simulink model "reaction_pendulum_swingup"  (R2021b)
settings: Solver=FixedStepDiscrete  StartTime=0.0  StopTime=15  FixedStep=h  RelTol=1e-3  EnableMultiTasking=on
PreLoadFcn:
  | warning('off','MATLAB:dispatcher:InexactMatch');
InitFcn:
  | startup_sequence
StartFcn:
  | startup_sequence
model workspace (MAT data in the model file):
  square_freq = 0.5
values from neighbouring files (symbols this model uses):
  F = A22-L*A12    [Reduced_observer.m]
  G = A21-L*A11+F*L    [Reduced_observer.m]
  H = B2-L*B1    [Reduced_observer.m]
  K_LQR = lqr(A,B,Q,R)    [LQR_gain.m]
  L = 10    [LQR_gain.m]    (also in Reduced_observer.m = place(A22',A12',pole)')
  linearization_point = [pi;0;0]    [startup_sequence.m]
  lp_deviation = [deg2rad((rand()-0.5)*50+180);0;0]    [startup_sequence.m]
undefined symbols (not defined in the file or in its folder): DiscIntNeverNeededParam, H_nlobs
settings Model: ExtModeTrigDuration=100000  Creator=user  LastModifiedBy=niels
settings DataIOCC: SaveFormat=Array  SignalLoggingSaveFormat=ModelDataLogs  SaveOutput=off  SignalLogging=off  DSMLogging=off  SaveTime=off  ReturnWorkspaceOutputs=off
settings OptimizationCC: ExpressionDepthLimit=2147483647  LifeSpan=inf
settings DebuggingCC: UnderspecifiedInitializationDetection=Classic  MergeDetectMultiDrivingBlocksExec=none  SolverPrmCheckMsg=warning  FcnCallInpInsideContextMsg=warning  StateNameClashWarn=warning  SFUnexpectedBacktrackingDiag=warning  SFNoUnconditionalDefaultTransitionDiag=warning  SFExecutionAtInitializationDiag=none  ArithmeticOperatorsInVariantConditions=warning
settings HardwareCC: ProdBitPerPointer=32  ProdBitPerSizeT=32  ProdBitPerPtrDiffT=32  ProdLargestAtomicFloat=None  ProdIntDivRoundTo=Undefined  ProdEndianess=Unspecified  ProdWordSize=32  ProdHWDeviceType=32-bit Generic
settings ModelReferenceCC: PropagateSignalLabelsOutOfModel=off
settings SFSimCC: SimUseLocalCustomCode=off  CustomCodeUndefinedFunction=UseInterfaceOnly
settings RTWCC: Description=rpend RTDAC/USB2 (Visual C/C++)  SystemTargetFile=rtcon_rpend_usb2.tlc  TemplateMakefile=rtcon_rpend_vc_usb2_x64.tmf  RTWUseLocalCustomCode=off
settings CodeAppCC: StateflowObjectComments=on
settings STFCustomTargetCC: ModelReferenceCompliant=off  CombineOutputUpdateFcns=on  MatFileLogging=on  GRTInterface=off  SystemTargetFile=rtcon_rpend_usb2.tlc
settings GRTTargetCC: TargetLangStandard=C89/C90 (ANSI)  ModelReferenceCompliant=off  ParMdlRefBuildCompliant=off  CompOptLevelCompliant=off  ConcurrentExecutionCompliant=off  CPPClassGenCompliant=off  UseToolchainInfoCompliant=off  ExtMode=on  ExtModeMexFile=rtcon_ext_comm
settings ConfigComp: CovMetricSettings=dw  CovSaveCumulativeToWorkspaceVar=on  CovSaveSingleToWorkspaceVar=on  CovExternalEMLEnable=off  CovSFcnEnable=off

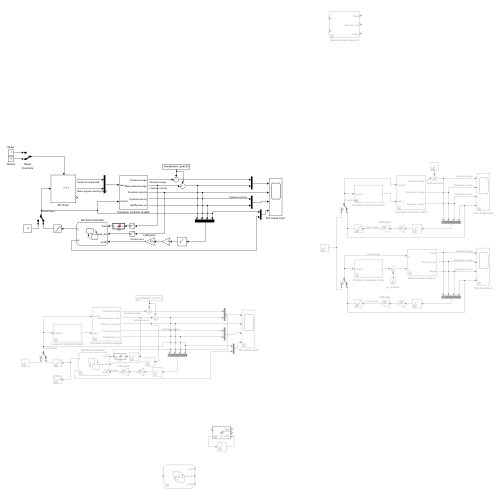
[thumbnail: Simulink's stored preview of the top-level diagram]
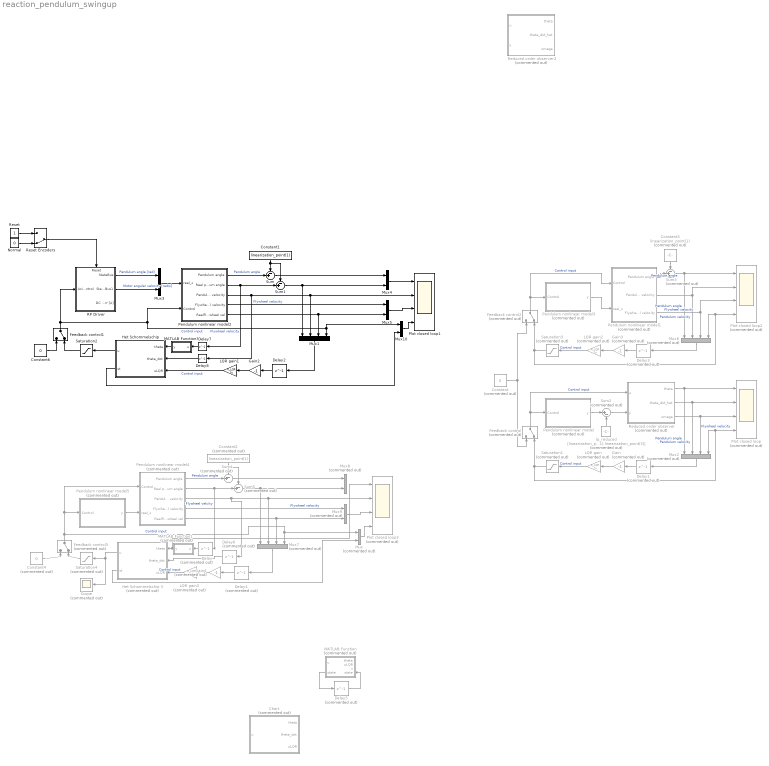
== system reaction_pendulum_swingup ==
  Chart : Stateflow chart  Commented=on  TreatAsAtomicUnit=on
  Constant : Constant  Commented=on  Value=0
  Constant1 : Constant  Value=linearization_point(1)
  Constant2 : Constant  Commented=on  Value=linearization_point(1)
  Constant3 : Constant  Commented=on  Value=linearization_point(1)
  Constant4 : Constant  Commented=on  Value=0
  Constant6 : Constant  Value=0
  Delay{,1,3..6} (6 alike) : Delay  Commented=on  DelayLength=1
  Delay2 : Delay  DelayLength=1
  Delay7 : Delay  DelayLength=1
  Delay8 : Delay  DelayLength=1
  Feedback control : ManualSwitch  Commented=on  CurrentSetting=0
  Feedback control1 : ManualSwitch  CurrentSetting=0
  Feedback control2 : ManualSwitch  Commented=on  CurrentSetting=0
  Feedback control3 : ManualSwitch  Commented=on  CurrentSetting=0
  Gain : Gain  Commented=on  Gain=-1
  Gain2 : Gain  Gain=-1
  Gain3 : Gain  Commented=on  Gain=-1
  Gain4 : Gain  Commented=on  Gain=-1
  Het Schommelschip : Stateflow chart  TreatAsAtomicUnit=on
  Het Schommelschip 3 : Stateflow chart  Commented=on  TreatAsAtomicUnit=on
  LQR gain : Gain  Commented=on  Gain=K_LQR  Multiplication=Matrix(K*u)
  LQR gain1 : Gain  Gain=K_LQR  Multiplication=Matrix(K*u)
  LQR gain2 : Gain  Commented=on  Gain=K_LQR  Multiplication=Matrix(K*u)
  LQR gain3 : Gain  Commented=on  Gain=K_LQR  Multiplication=Matrix(K*u)
  MATLAB Function : MATLAB Function  Commented=on  TreatAsAtomicUnit=on
  MATLAB Function1 : MATLAB Function  Commented=on  TreatAsAtomicUnit=on
  MATLAB Function3 : MATLAB Function  TreatAsAtomicUnit=on
  Mux : Mux  Commented=on  Inputs=2
  Mux1 : Mux
  Mux{3..5,10} (4 alike) : Mux  Inputs=2
  Mux2 : Mux  Commented=on
  Mux6 : Mux  Commented=on
  Mux7 : Mux  Commented=on
  Mux8 : Mux  Commented=on  Inputs=2
  Mux9 : Mux  Commented=on  Inputs=2
  Normal : Constant  Value=0
  Pendulum nonlinear model : Subsystem  Commented=on
  Pendulum nonlinear model1 : Subsystem  Commented=on
  Pendulum nonlinear model2 : Subsystem
  Pendulum nonlinear model3 : Subsystem  Commented=on
  Pendulum nonlinear model4 : Subsystem  Commented=on
  Pendulum nonlinear model5 : Subsystem  Commented=on
  Plot closed loop : Scope  Commented=on  NumInputPorts=4
  Plot closed loop1 : Scope  NumInputPorts=4
  Plot closed loop2 : Scope  Commented=on  NumInputPorts=4
  Plot closed loop3 : Scope  Commented=on  NumInputPorts=4
  RP Driver : Subsystem
      settings: PortSchema="{\"entries\":[{\"content\":{\"sides\":[{\"content\":{\"connectorIds\":[\"In1\"]},\"type\":\"ConnectorPlacement.EquallySpacedRectSide\",\"uuid\":\"28df0a7f-6242-4d39-ac1c-ff3ee0c6a4e1\"},{\"content\":{\"connectorIds\":[\"Out1\",\"Out2\",\"Out3\"],\"side\":\"RIGHT\"},\"type\":\"ConnectorPlacement.EquallySpacedRectSide\",\"uuid\":\"435de4ce-8687-493c-bad7-12ebb99ee6db\"},{\"content\":{\"connectorIds\":[\"In2\"],\"side\":\"TOP\"},\"type\":\"ConnectorPlacement.EquallySpacedRectSide\",\"uuid\":\"946ce8c1-4b6f-49e8-9b13-de0bfa90dc27\"},{\"content\":{\"side\":\"BOTTOM\"},\"type\":\"ConnectorPlacement.EquallySpacedRectSide\",\"uuid\":\"2521f2e0-71e2-448f-85b3-c4d5eb7ca065\"}]},\"type\":\"ConnectorPlacement.EquallySpacedConnector\",\"uuid\":\"0b989423-35e3-4087-b06d-cef0c97f9c21\"}],\"packageUris\":[\"http://schema.mathworks.com/mf0/Connector/R2020b\"],\"version\":\"1.0\"}"
      mask Display: image(imread('rwp.JPG'))
  Reduced order observer : Subsystem  Commented=on
  Reduced order observer2 : Subsystem  Commented=on
  Reset : Constant
  Reset Encoders : ManualSwitch  CurrentSetting=0
  Saturation1 : Saturate  Commented=on  UpperLimit=1  LowerLimit=-1
  Saturation2 : Saturate  UpperLimit=1  LowerLimit=-1
  Saturation3 : Saturate  Commented=on  UpperLimit=1  LowerLimit=-1
  Saturation4 : Saturate  Commented=on  UpperLimit=1  LowerLimit=-1
  Scope : Scope  Commented=on
  Sum : Sum  Inputs=-+|
  Sum1 : Sum  Inputs=-+|
  Sum2 : Sum  Commented=on  Inputs=|+-
  Sum3 : Sum  Commented=on  Inputs=-+|
  Sum4 : Sum  Commented=on  Inputs=-+|
  Sum5 : Sum  Commented=on  Inputs=-+|
  lp_reduced : Constant  Commented=on  Value=[linearization_point(1);linearization_point(3)]
  wires:
  Normal/1 -> Reset Encoders/2
  Reset/1 -> Reset Encoders/1
  Reset Encoders/1 -> RP Driver/2(Reset)
  RP Driver/1(StateBus) -> Mux3/1  "Pendulum angle [rad]"
  Feedback control/1 -> Reduced order observer/1(u), Pendulum nonlinear model/1(Control)  "Control input"
  LQR gain/1 -> Saturation1/1  "Control input"
  Gain/1 -> LQR gain/1
  Delay1/1 -> Gain/1
  Reduced order observer/2(theta_dot_hat) -> Plot closed loop/2, Mux2/2  "Pendulum velocity"
  Sum2/1 -> Reduced order observer/2(y)
  lp_reduced/1 -> Sum2/2
  Pendulum nonlinear model/1(y) -> Sum2/1
  Reduced order observer/1(theta) -> Plot closed loop/1, Mux2/1  "Pendulum angle"
  Reduced order observer/3(omega) -> Plot closed loop/3, Mux2/3  "Flywheel velocity"
  Mux2/1 -> Delay1/1
  Mux1/1 -> Delay2/1
  Gain2/1 -> LQR gain1/1
  Delay2/1 -> Gain2/1
  Feedback control1/1 -> Pendulum nonlinear model2/2(Control), Mux10/1, Mux1/4, RP Driver/1(Azimuth Control)  "Control input"
  Saturation2/1 -> Feedback control1/2
  Saturation1/1 -> Plot closed loop/4, Mux2/4, Feedback control/2
  Constant1/1 -> Sum1/1, Sum/1
  Mux4/1 -> Plot closed loop1/1
  Mux5/1 -> Plot closed loop1/3
  Sum1/1 -> Mux4/2, Mux1/1
  Pendulum nonlinear model1/1(Pendulum angle) -> Sum3/2  "Pendulum angle"
  Constant3/1 -> Sum3/1
  Saturation3/1 -> Plot closed loop2/4, Mux6/4, Feedback control2/2
  Pendulum nonlinear model3/1(y) -> Pendulum nonlinear model1/2(real_x)
  Sum3/1 -> Plot closed loop2/1, Mux6/1  "Pendulum angle"
  Gain3/1 -> LQR gain2/1
  Pendulum nonlinear model1/2(Pendulum velocity) -> Plot closed loop2/2, Mux6/2  "Pendulum velocity"
  LQR gain2/1 -> Saturation3/1  "Control input"
  Pendulum nonlinear model1/3(Flywheel velocity) -> Plot closed loop2/3, Mux6/3  "Flywheel velocity"
  Mux6/1 -> Delay3/1
  Delay3/1 -> Gain3/1
  Feedback control2/1 -> Pendulum nonlinear model3/1(Control), Pendulum nonlinear model1/1(Control)  "Control input"
  Constant/1 -> Feedback control/1, Feedback control2/1
  Delay4/1 -> Gain4/1
  Feedback control3/1 -> Pendulum nonlinear model4/1(Control), Pendulum nonlinear model5/1(Control), Mux/1, Mux7/4  "Control input"
  Gain4/1 -> LQR gain3/1
  Pendulum nonlinear model5/1(y) -> Pendulum nonlinear model4/2(real_x)
  Constant4/1 -> Feedback control3/1
  Constant6/1 -> Feedback control1/1
  RP Driver/2(StateBus1) -> Mux3/2  "Motor angular velocity [rad/s]"
  Sum/1 -> Mux4/1
  Sum4/1 -> Mux8/1
  Pendulum nonlinear model4/4(Flywheel velocity) -> Mux9/1  "Flywheel velocity"
  Saturation4/1 -> Feedback control3/2
  Pendulum nonlinear model4/5(Realflywheel vel) -> Mux7/3, Mux9/2
  Mux9/1 -> Plot closed loop3/3
  Sum5/1 -> Mux8/2, Mux7/1
  Pendulum nonlinear model4/1(Pendulum angle) -> Sum4/2  "Pendulum angle"
  Constant2/1 -> Sum5/1, Sum4/1
  Mux7/1 -> Delay4/1
  Pendulum nonlinear model4/3(Pendulum velocity) -> Delay6/1, Mux7/2, Plot closed loop3/2
  Pendulum nonlinear model4/2(Real pendulum angle) -> Sum5/2, Delay/1  "Flywheel velcity"
  Pendulum nonlinear model2/1(Pendulum angle) -> Sum/2  "Pendulum angle"
  Pendulum nonlinear model2/2(Real pendulum angle) -> Delay7/1, Sum1/2  "Flywheel velocity"
  Pendulum nonlinear model2/3(Pendulum velocity) -> Delay8/1, Mux1/2, Plot closed loop1/2
  Pendulum nonlinear model2/4(Flywheel velocity) -> Mux5/1  "Flywheel velocity"
  Pendulum nonlinear model2/5(Realflywheel vel) -> Mux5/2, Mux1/3
  Mux3/1 -> Pendulum nonlinear model2/1(real_x)
  Delay5/1 -> MATLAB Function/4("state ")
  MATLAB Function/2(state) -> Delay5/1
  LQR gain3/1 -> Het Schommelschip 3/3(uLQR)  "Control input"
  Het Schommelschip 3/1(u) -> Scope/1, Saturation4/1
  Delay6/1 -> Het Schommelschip 3/2(theta_dot)
  Delay/1 -> MATLAB Function1/1(u)
  MATLAB Function1/1(y) -> Plot closed loop3/1, Het Schommelschip 3/1(theta)
  MATLAB Function3/1(y) -> Het Schommelschip/1(theta)
  Delay8/1 -> Het Schommelschip/2(theta_dot)
  Delay7/1 -> MATLAB Function3/1(u)
  LQR gain1/1 -> Het Schommelschip/3(uLQR)  "Control input"
  Mux/1 -> Plot closed loop3/4
  Het Schommelschip 3/2(st) -> Mux/2
  Het Schommelschip/1(u) -> Saturation2/1
  Mux10/1 -> Plot closed loop1/4
  Het Schommelschip/2(st) -> Mux10/2

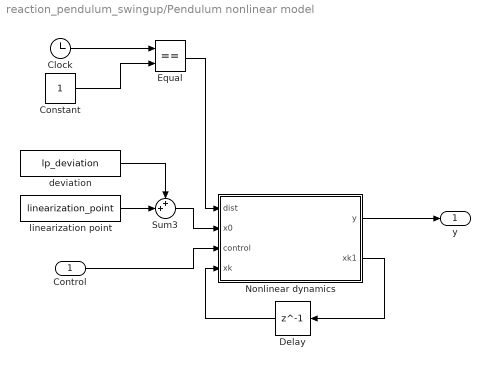
== system reaction_pendulum_swingup/Pendulum nonlinear model ==
  Control : Inport
  Clock : Clock
  Constant : Constant
  Delay : Delay  DelayLength=1
  Equal : RelationalOperator  Operator===  OutDataTypeStr=boolean  RndMeth=Simplest
  Nonlinear dynamics : MATLAB Function  TreatAsAtomicUnit=on
  Sum3 : Sum  Inputs=++|
  deviation : Constant  Value=lp_deviation
  linearization point : Constant  Value=linearization_point
  y : Outport
  wires:
  Delay/1 -> Nonlinear dynamics/4(xk)
  Sum3/1 -> Nonlinear dynamics/2(x0)
  Control/1 -> Nonlinear dynamics/3(control)
  Nonlinear dynamics/2(xk1) -> Delay/1
  Nonlinear dynamics/1(y) -> y/1
  deviation/1 -> Sum3/1
  linearization point/1 -> Sum3/2
  Constant/1 -> Equal/2
  Equal/1 -> Nonlinear dynamics/1(dist)
  Clock/1 -> Equal/1

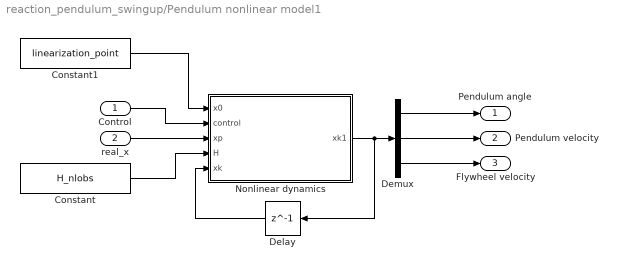
== system reaction_pendulum_swingup/Pendulum nonlinear model1 ==
  Control : Inport
  real_x : Inport  Port=2
  Constant : Constant  Value=H_nlobs
  Constant1 : Constant  Value=linearization_point
  Delay : Delay  DelayLength=1
  Demux : Demux  Outputs=3
  Nonlinear dynamics : MATLAB Function  TreatAsAtomicUnit=on
  Pendulum angle : Outport
  Pendulum velocity : Outport  Port=2
  Flywheel velocity : Outport  Port=3
  wires:
  Delay/1 -> Nonlinear dynamics/5(xk)
  Control/1 -> Nonlinear dynamics/2(control)
  Nonlinear dynamics/1(xk1) -> Demux/1, Delay/1
  real_x/1 -> Nonlinear dynamics/3(xp)
  Constant/1 -> Nonlinear dynamics/4(H)
  Constant1/1 -> Nonlinear dynamics/1(x0)
  Demux/2 -> Pendulum velocity/1
  Demux/1 -> Pendulum angle/1
  Demux/3 -> Flywheel velocity/1

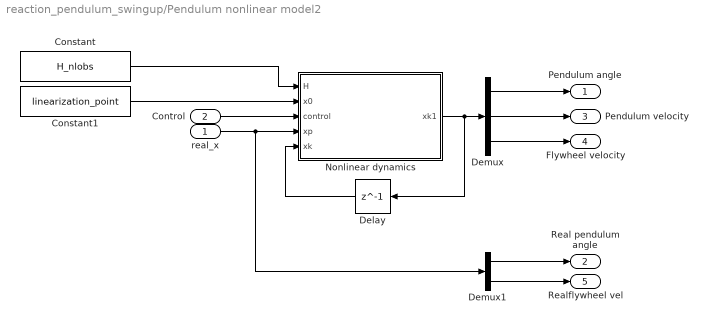
== system reaction_pendulum_swingup/Pendulum nonlinear model2 ==
  real_x : Inport
  Control : Inport  Port=2
  Constant : Constant  Value=H_nlobs
  Constant1 : Constant  Value=linearization_point
  Delay : Delay  DelayLength=1
  Demux : Demux  Outputs=3
  Demux1 : Demux  Outputs=2
  Nonlinear dynamics : MATLAB Function  TreatAsAtomicUnit=on
  Pendulum angle : Outport
  Real pendulum angle : Outport  Port=2
  Pendulum velocity : Outport  Port=3
  Flywheel velocity : Outport  Port=4
  Realflywheel vel : Outport  Port=5
  wires:
  Delay/1 -> Nonlinear dynamics/5(xk)
  Control/1 -> Nonlinear dynamics/3(control)
  Nonlinear dynamics/1(xk1) -> Demux/1, Delay/1
  real_x/1 -> Demux1/1, Nonlinear dynamics/4(xp)
  Constant/1 -> Nonlinear dynamics/1(H)
  Constant1/1 -> Nonlinear dynamics/2(x0)
  Demux/2 -> Pendulum velocity/1
  Demux/1 -> Pendulum angle/1
  Demux/3 -> Flywheel velocity/1
  Demux1/1 -> Real pendulum angle/1
  Demux1/2 -> Realflywheel vel/1

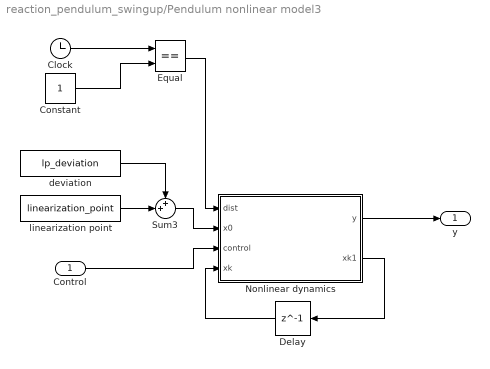
== system reaction_pendulum_swingup/Pendulum nonlinear model3 ==
  Control : Inport
  Clock : Clock
  Constant : Constant
  Delay : Delay  DelayLength=1
  Equal : RelationalOperator  Operator===  OutDataTypeStr=boolean  RndMeth=Simplest
  Nonlinear dynamics : MATLAB Function  TreatAsAtomicUnit=on
  Sum3 : Sum  Inputs=++|
  deviation : Constant  Value=lp_deviation
  linearization point : Constant  Value=linearization_point
  y : Outport
  wires:
  Delay/1 -> Nonlinear dynamics/4(xk)
  Sum3/1 -> Nonlinear dynamics/2(x0)
  Control/1 -> Nonlinear dynamics/3(control)
  Nonlinear dynamics/2(xk1) -> Delay/1
  Nonlinear dynamics/1(y) -> y/1
  deviation/1 -> Sum3/1
  linearization point/1 -> Sum3/2
  Clock/1 -> Equal/1
  Constant/1 -> Equal/2
  Equal/1 -> Nonlinear dynamics/1(dist)

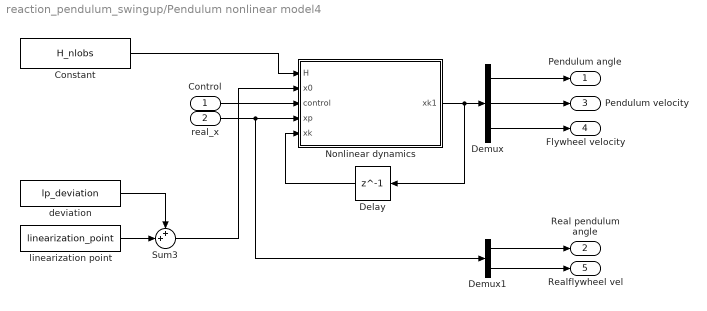
== system reaction_pendulum_swingup/Pendulum nonlinear model4 ==
  Control : Inport
  real_x : Inport  Port=2
  Constant : Constant  Value=H_nlobs
  Delay : Delay  DelayLength=1
  Demux : Demux  Outputs=3
  Demux1 : Demux  Outputs=2
  Nonlinear dynamics : MATLAB Function  TreatAsAtomicUnit=on
  Sum3 : Sum  Inputs=++|
  deviation : Constant  Value=lp_deviation
  linearization point : Constant  Value=linearization_point
  Pendulum angle : Outport
  Real pendulum angle : Outport  Port=2
  Pendulum velocity : Outport  Port=3
  Flywheel velocity : Outport  Port=4
  Realflywheel vel : Outport  Port=5
  wires:
  Delay/1 -> Nonlinear dynamics/5(xk)
  Control/1 -> Nonlinear dynamics/3(control)
  Nonlinear dynamics/1(xk1) -> Demux/1, Delay/1
  real_x/1 -> Demux1/1, Nonlinear dynamics/4(xp)
  Constant/1 -> Nonlinear dynamics/1(H)
  Sum3/1 -> Nonlinear dynamics/2(x0)
  Demux/2 -> Pendulum velocity/1
  Demux/1 -> Pendulum angle/1
  Demux/3 -> Flywheel velocity/1
  Demux1/1 -> Real pendulum angle/1
  Demux1/2 -> Realflywheel vel/1
  linearization point/1 -> Sum3/2
  deviation/1 -> Sum3/1

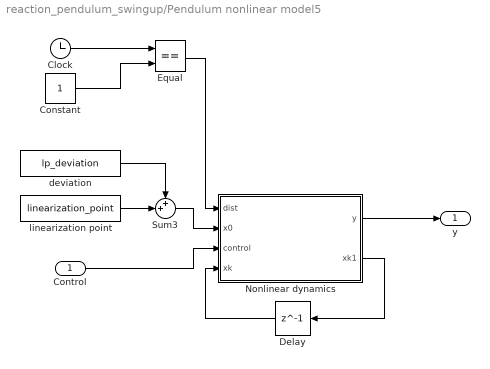
== system reaction_pendulum_swingup/Pendulum nonlinear model5 ==
  Control : Inport
  Clock : Clock
  Constant : Constant
  Delay : Delay  DelayLength=1
  Equal : RelationalOperator  Operator===  OutDataTypeStr=boolean  RndMeth=Simplest
  Nonlinear dynamics : MATLAB Function  TreatAsAtomicUnit=on
  Sum3 : Sum  Inputs=++|
  deviation : Constant  Value=lp_deviation
  linearization point : Constant  Value=linearization_point
  y : Outport
  wires:
  Delay/1 -> Nonlinear dynamics/4(xk)
  Sum3/1 -> Nonlinear dynamics/2(x0)
  Control/1 -> Nonlinear dynamics/3(control)
  Nonlinear dynamics/2(xk1) -> Delay/1
  Nonlinear dynamics/1(y) -> y/1
  deviation/1 -> Sum3/1
  linearization point/1 -> Sum3/2
  Clock/1 -> Equal/1
  Constant/1 -> Equal/2
  Equal/1 -> Nonlinear dynamics/1(dist)

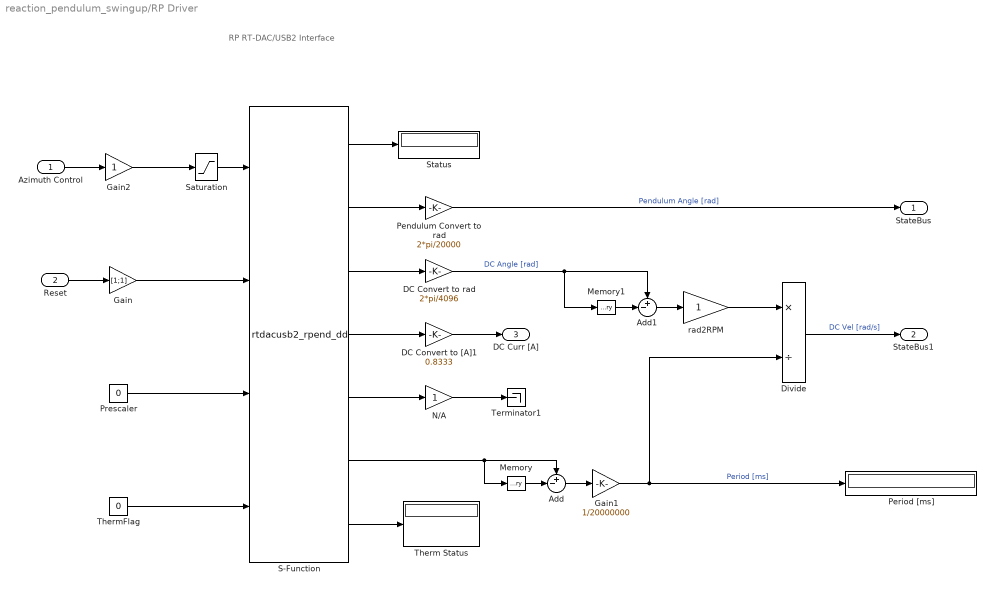
== system reaction_pendulum_swingup/RP Driver ==
  note: RP RT-DAC/USB2
      | Interface
  Azimuth Control : Inport
  Reset : Inport  Port=2
  Add : Sum  Inputs=+-|
  Add1 : Sum  Inputs=+-|
  DC Convert to [A]1 : Gain  Gain=0.8333  SaturateOnIntegerOverflow=on  OutDataTypeStr=Inherit: Same as input  ParamDataTypeStr=Inherit: Same as input
  DC Convert to rad : Gain  Gain=2*pi/4096  SaturateOnIntegerOverflow=on  OutDataTypeStr=Inherit: Same as input  ParamDataTypeStr=Inherit: Same as input
  Divide : Product  Inputs=*/
  Gain : Gain  Gain=[1;1]
  Gain1 : Gain  Gain=1/20000000
  Gain2 : Gain
  Memory : Memory
  Memory1 : Memory
  N/A : Gain  SaturateOnIntegerOverflow=on  OutDataTypeStr=Inherit: Same as input  ParamDataTypeStr=Inherit: Same as input
  Pendulum Convert to rad : Gain  Gain=2*pi/20000  SaturateOnIntegerOverflow=on  OutDataTypeStr=Inherit: Same as input  ParamDataTypeStr=Inherit: Same as input
  Period [ms] : Display
  Prescaler : Constant  Value=0
  S-Function : S-Function  FunctionName=rtdacusb2_rpend_dd  Parameters=1, h  SFunctionDeploymentMode=off  EnableBusSupport=off
  Saturation : Saturate  UpperLimit=1  LowerLimit=-1
  Status : Display
  Terminator1 : Terminator
  Therm Status : Display
  ThermFlag : Constant  Value=0
  rad2RPM : Gain  SaturateOnIntegerOverflow=on  OutDataTypeStr=Inherit: Same as input  ParamDataTypeStr=Inherit: Same as input
  StateBus : Outport  VectorParamsAs1DForOutWhenUnconnected=off
  StateBus1 : Outport  Port=2  VectorParamsAs1DForOutWhenUnconnected=off
  DC Curr [A] : Outport  Port=3  VectorParamsAs1DForOutWhenUnconnected=off
  wires:
  S-Function/7 -> Therm Status/1
  S-Function/5 -> N/A/1
  S-Function/4 -> DC Convert to [A]1/1
  ThermFlag/1 -> S-Function/4
  Prescaler/1 -> S-Function/3
  Gain/1 -> S-Function/2
  DC Convert to [A]1/1 -> DC Curr [A]/1
  Divide/1 -> StateBus1/1  "DC Vel [rad/s]"
  rad2RPM/1 -> Divide/1
  Add1/1 -> rad2RPM/1
  Memory1/1 -> Add1/2
  N/A/1 -> Terminator1/1
  S-Function/6 -> Add/1, Memory/1
  Gain2/1 -> Saturation/1
  Gain1/1 -> Period [ms]/1, Divide/2  "Period [ms]"
  Add/1 -> Gain1/1
  Memory/1 -> Add/2
  DC Convert to rad/1 -> Add1/1, Memory1/1  "DC Angle [rad]"
  S-Function/3 -> DC Convert to rad/1
  Pendulum Convert to rad/1 -> StateBus/1  "Pendulum Angle [rad]"
  S-Function/2 -> Pendulum Convert to rad/1
  S-Function/1 -> Status/1
  Saturation/1 -> S-Function/1
  Reset/1 -> Gain/1
  Azimuth Control/1 -> Gain2/1

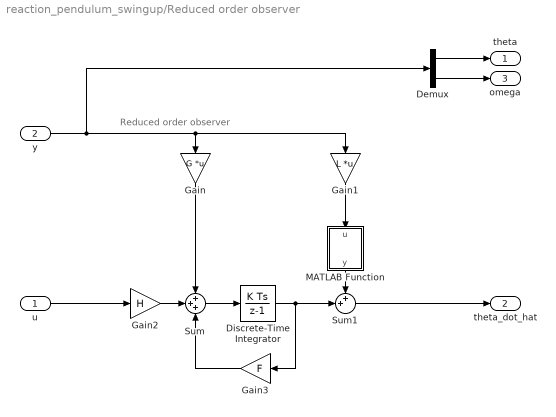
== system reaction_pendulum_swingup/Reduced order observer ==
  note: Reduced order observer
  u : Inport
  y : Inport  Port=2
  Demux : Demux  Outputs=2
  Discrete-Time Integrator : DiscreteIntegrator  SampleTime=-1  ICPrevOutput=DiscIntNeverNeededParam  ICPrevScaledInput=DiscIntNeverNeededParam
  Gain : Gain  Gain=G  Multiplication=Matrix(K*u)
  Gain1 : Gain  Gain=L  Multiplication=Matrix(K*u)
  Gain2 : Gain  Gain=H
  Gain3 : Gain  Gain=F
  MATLAB Function : MATLAB Function  TreatAsAtomicUnit=on
  Sum : Sum  Inputs=+++
  Sum1 : Sum  Inputs=++|
  theta : Outport
  theta_dot_hat : Outport  Port=2
  omega : Outport  Port=3
  wires:
  u/1 -> Gain2/1
  Gain2/1 -> Sum/2
  Gain/1 -> Sum/1
  Sum/1 -> Discrete-Time Integrator/1
  Discrete-Time Integrator/1 -> Gain3/1, Sum1/2
  Gain3/1 -> Sum/3
  Sum1/1 -> theta_dot_hat/1
  y/1 -> Gain1/1, Gain/1, Demux/1
  Demux/1 -> theta/1
  Demux/2 -> omega/1
  Gain1/1 -> MATLAB Function/1(u)
  MATLAB Function/1(y) -> Sum1/1

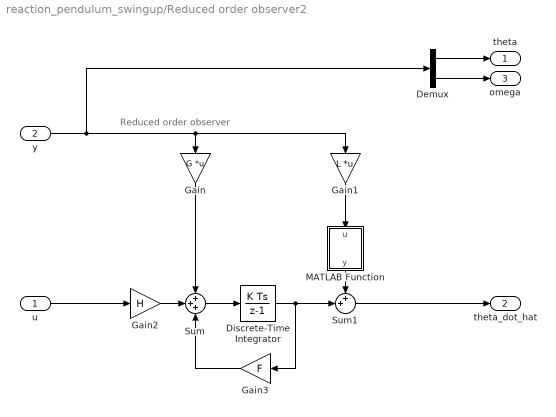
== system reaction_pendulum_swingup/Reduced order observer2 ==
  note: Reduced order observer
  u : Inport
  y : Inport  Port=2
  Demux : Demux  Outputs=2
  Discrete-Time Integrator : DiscreteIntegrator  SampleTime=-1  ICPrevOutput=DiscIntNeverNeededParam  ICPrevScaledInput=DiscIntNeverNeededParam
  Gain : Gain  Gain=G  Multiplication=Matrix(K*u)
  Gain1 : Gain  Gain=L  Multiplication=Matrix(K*u)
  Gain2 : Gain  Gain=H
  Gain3 : Gain  Gain=F
  MATLAB Function : MATLAB Function  TreatAsAtomicUnit=on
  Sum : Sum  Inputs=+++
  Sum1 : Sum  Inputs=++|
  theta : Outport
  theta_dot_hat : Outport  Port=2
  omega : Outport  Port=3
  wires:
  u/1 -> Gain2/1
  Gain2/1 -> Sum/2
  Gain/1 -> Sum/1
  Sum/1 -> Discrete-Time Integrator/1
  Discrete-Time Integrator/1 -> Gain3/1, Sum1/2
  Gain3/1 -> Sum/3
  Sum1/1 -> theta_dot_hat/1
  y/1 -> Gain1/1, Gain/1, Demux/1
  Demux/1 -> theta/1
  Demux/2 -> omega/1
  Gain1/1 -> MATLAB Function/1(u)
  MATLAB Function/1(y) -> Sum1/1

== matlab function reaction_pendulum_swingup/Reduced order observer2/MATLAB Function ==
  data: u input; y output
function y = fcn(u)
    persistent obs_init
    y=u;
    if isempty(obs_init)
        y=0;
        obs_init = true;
    end
end

== matlab function reaction_pendulum_swingup/Pendulum nonlinear model3/Nonlinear dynamics ==
  data: dist input; x0 input; y output; control input; xk input size=[3,1]; xk1 output size=[3,1]; h parameter
function [y, xk1] = nlrk4(dist, x0, control, xk, h)
    persistent initialized

    if isempty(initialized)
        xk = x0;
        initialized = true;
    end

    function dx = nlf(t,x,u)
    
        % Define constants
        K1 = 10.6608;
        K2 = 0.0487;
        K3 = 0.1031;
        K4 = 404.3827;
        K5 = 0.9442;
        K6 = 1.7125;
        K_tau = 0.0107;
        
        % System equations
        theta = x(1);
        theta_dot = x(2);
        omega = x(3);
        theta_ddot = -K1*sin(theta)-K2*theta_dot-K3*sign(theta_dot)-K_tau*(K4*u-K5*omega-K6*sign(omega));
        omega_dot = K4*u-K5*omega-K6*sign(omega);
        dx = [theta_dot; theta_ddot; omega_dot];
    end

    % Executes one timestep of the RK4 algorithm
    k1 = nlf(0, xk, control);
    k2 = nlf(0 + h/2, xk + h/2*k1, control);
    k3 = nlf(0 + h/2, xk + h/2*k2, control);
    k4 = nlf(0 + h, xk + h*k3, control);
    xk1 = xk + h/6*(k1 + 2*k2 + 2*k3 + k4);
    
    if dist
        xk1(1)=pi+deg2rad(5);
        xk(1) =pi+deg2rad(5);
    end

    % % Forward Euler
    % xk1 = xk + h*nlf(0, xk, control);
    % Take out states of interest
    y = [xk(1); xk(3)];
end

== matlab function reaction_pendulum_swingup/Pendulum nonlinear model4/Nonlinear dynamics ==
  data: H input; x0 input; control input; xp input; xk input size=[3,1]; xk1 output size=[3,1]; h parameter
function xk1   = nlrk4(H, x0, control, xp, xk, h)
    persistent initialized

    if isempty(initialized)
        xk1 = x0;
        theta_dd = 0;
        initialized = true;
        return;
    end

    function dx = nlf(t,x,u,xp,H)
        C = [1,0,0;0,0,1];

        % Define constants
        K1 = 10.6608;
        K2 = 0.0487;
        K3 = 0.1031;
        K4 = 404.3827;
        K5 = 0.9442;
        K6 = 1.7125;
        K_tau = 0.0107;
        
        % System equations
        theta = x(1);
        theta_dot = x(2);
        omega = x(3);
        theta_ddot = -K1*sin(theta)-K2*theta_dot-K3*sign(theta_dot)-K_tau*(K4*u-K5*omega-K6*sign(omega));
        omega_dot = K4*u-K5*omega-K6*sign(omega);
        delta = xp-C*x;
        Linear_term = H*(delta);
        NL_term = [theta_dot; theta_ddot; omega_dot] ;
        dx = NL_term + Linear_term;
    end

    function theta_ddot = theta_ddd(t,x,u,xp,H)
        C = [1,0,0;0,0,1];

        % Define constants
        K1 = 10.6608;
        K2 = 0.0487;
        K3 = 0.1031;
        K4 = 404.3827;
        K5 = 0.9442;
        K6 = 1.7125;
        K_tau = 0.0107;
        
        % System equations
        theta = x(1);
        theta_dot = x(2);
        omega = x(3);
        theta_ddot = -K1*sin(theta)-K2*theta_dot-K3*sign(theta_dot)-K_tau*(K4*u-K5*omega-K6*sign(omega));
    end

    theta_dd = theta_ddd(0, xk, control, xp, H);

    % Executes one timestep of the RK4 algorithm
    k1 = nlf(0, xk, control, xp, H);
    k2 = nlf(0 + h/2, xk + h/2*k1, control, xp + h/2*k1([1,3]), H);
    k3 = nlf(0 + h/2, xk + h/2*k2, control, xp + h/2*k2([1,3]), H);
    k4 = nlf(0 + h, xk + h*k3, control, xp + h*k3([1,3]), H);
    xk1 = xk + h/6*(k1 + 2*k2 + 2*k3 + k4);

    % % Forward Euler
    % xk1 = xk + h*nlf(0, xk, control);
    % Take out states of interest
    % y = [xk(1); xk(3)];
end

== matlab function reaction_pendulum_swingup/Pendulum nonlinear model5/Nonlinear dynamics ==
  data: dist input; x0 input; y output; control input; xk input size=[3,1]; xk1 output size=[3,1]; h parameter
function [y, xk1] = nlrk4(dist, x0, control, xk, h)
    persistent initialized

    if isempty(initialized)
        xk = x0;
        initialized = true;
    end

    function dx = nlf(t,x,u)
    
        % Define constants
        K1 = 10.6608;
        K2 = 0.0487;
        K3 = 0.1031;
        K4 = 404.3827;
        K5 = 0.9442;
        K6 = 1.7125;
        K_tau = 0.0107;
        
        % System equations
        theta = x(1);
        theta_dot = x(2);
        omega = x(3);
        theta_ddot = -K1*sin(theta)-K2*theta_dot-K3*sign(theta_dot)-K_tau*(K4*u-K5*omega-K6*sign(omega));
        omega_dot = K4*u-K5*omega-K6*sign(omega);
        dx = [theta_dot; theta_ddot; omega_dot];
    end

    % Executes one timestep of the RK4 algorithm
    k1 = nlf(0, xk, control);
    k2 = nlf(0 + h/2, xk + h/2*k1, control);
    k3 = nlf(0 + h/2, xk + h/2*k2, control);
    k4 = nlf(0 + h, xk + h*k3, control);
    xk1 = xk + h/6*(k1 + 2*k2 + 2*k3 + k4);

    % if dist
    %     xk1(1)=pi/9;
    %     xk(1) = pi/9;
    % end

    % % Forward Euler
    % xk1 = xk + h*nlf(0, xk, control);
    % Take out states of interest
    y = [xk(1); xk(3)];
end

== matlab function reaction_pendulum_swingup/MATLAB Function ==
  data: theta input; uLQR input; x input; u output; state input; state output
function [u, state] = fcn(theta, uLQR, x, state)

u = zeros(1);

theta = mod(theta,2*pi);
theta_dot = x(2);

delta = deg2rad(25);
delta2 = deg2rad(55);

ku=0.4; % accelation constant
kp=1; % decelleration constant

if pi-delta < theta && theta < pi+delta 
    u = uLQR;
    disp("Stabilizing")
elseif pi-delta2 < theta && theta < pi+delta2 
    u = kp*sign(theta_dot);
    disp("Slowing down")
else
    u = -ku*sign(theta_dot);
    disp("Accelerating")
end

== stateflow chart reaction_pendulum_swingup/Chart ==
  state Swing_up
    u=-ku*sign(theta_dot);
  state Slow_down
    u=kp*sign(theta_dot);
  state Nothing2
    u=0;
  state Stabilizing
    u=uLQR;
  (default) -> Swing_up
  Nothing2 -> Swing_up [order 1] : [abs(theta_dot)<2]
  Swing_up -> Slow_down : [pi-delta2 < theta && theta < pi+delta2]
  Nothing2 -> Slow_down [order 2] : [pi-delta2 < theta && theta < pi+delta2]
  Slow_down -> Stabilizing [order 1] : [pi-delta < theta && theta < pi+delta && abs(theta_dot)<0.3]
  Slow_down -> Stabilizing [order 2] : [abs(theta_dot)<0.5]
  Stabilizing -> Nothing2 : [pi-delta2 > theta || theta > pi+delta2]
  data: theta input; theta_dot input; u output; ku local =0.4; kp local =1; delta local =deg2rad(15); delta2 local =deg2rad(32); uLQR input

== matlab function reaction_pendulum_swingup/MATLAB Function1 ==
  data: u input; y output
function y = fcn(u)

y = mod(u,2*pi)-pi;

end

== stateflow chart reaction_pendulum_swingup/Het Schommelschip ==
  state Swing_up
    u=-ku*sign(theta_dot);
    st = -0.1;
  state Nothing
    u=0;
    st = 0;
  state Slow_down
    u=kp*sign(theta_dot);
    st = 0.1;
  state Stabilizing
    u=uLQR;
    st=0.4;
  (default) -> Swing_up
  Nothing -> Swing_up [order 1] : [abs(theta)>wheel]
  Swing_up -> Nothing : [abs(theta)<wheel]
  Nothing -> Slow_down [order 3] : [abs(theta)<pi/2 && abs(theta_dot)>vmax]
  Slow_down -> Nothing : [abs(theta_dot)<vmax]
  Nothing -> Stabilizing [order 2] : [abs(theta) < delta]
  Stabilizing -> Nothing : [abs(theta) > delta]
  data: theta input; theta_dot input; u output; ku local =0.8; kp local =1; delta local =deg2rad(20); uLQR input; vmax local =5; wheel local =3*pi/4; st output

== stateflow chart reaction_pendulum_swingup/Het Schommelschip 3 ==
  state Swing_up
    u=-ku*sign(theta_dot);
    st = -0.1;
  state Nothing
    u=0;
    st = 0;
  state Slow_down
    u=kp*sign(theta_dot);
    st = 0.1;
  state Stabilizing
    u=uLQR;
    st=0.4;
  (default) -> Swing_up
  Nothing -> Swing_up [order 1] : [abs(theta)>wheel]
  Swing_up -> Nothing : [abs(theta)<wheel]
  Nothing -> Slow_down [order 3] : [abs(theta)<pi/2 && abs(theta_dot)>vmax]
  Slow_down -> Nothing : [abs(theta_dot)<vmax]
  Nothing -> Stabilizing [order 2] : [abs(theta) < delta]
  Stabilizing -> Nothing : [abs(theta) > delta]
  data: theta input; theta_dot input; u output; ku local =0.8; kp local =1; delta local =deg2rad(20); uLQR input; vmax local =5; wheel local =3*pi/4; st output

== matlab function reaction_pendulum_swingup/MATLAB Function3 ==
  data: u input; y output
function y = fcn(u)

y = mod(u,2*pi)-pi;

end

== matlab function reaction_pendulum_swingup/Reduced order observer/MATLAB Function ==
  data: u input; y output
function y = fcn(u)
    persistent obs_init
    y=u;
    if isempty(obs_init)
        y=0;
        obs_init = true;
    end
end

== matlab function reaction_pendulum_swingup/Pendulum nonlinear model/Nonlinear dynamics ==
  data: dist input; x0 input; y output; control input; xk input size=[3,1]; xk1 output size=[3,1]; h parameter
function [y, xk1] = nlrk4(dist, x0, control, xk, h)
    persistent initialized

    if isempty(initialized)
        xk = x0;
        initialized = true;
    end

    function dx = nlf(t,x,u)
    
        % Define constants
        K1 = 10.6608;
        K2 = 0.0487;
        K3 = 0.1031;
        K4 = 404.3827;
        K5 = 0.9442;
        K6 = 1.7125;
        K_tau = 0.0107;
        
        % System equations
        theta = x(1);
        theta_dot = x(2);
        omega = x(3);
        theta_ddot = -K1*sin(theta)-K2*theta_dot-K3*sign(theta_dot)-K_tau*(K4*u-K5*omega-K6*sign(omega));
        omega_dot = K4*u-K5*omega-K6*sign(omega);
        dx = [theta_dot; theta_ddot; omega_dot];
    end

    % Executes one timestep of the RK4 algorithm
    k1 = nlf(0, xk, control);
    k2 = nlf(0 + h/2, xk + h/2*k1, control);
    k3 = nlf(0 + h/2, xk + h/2*k2, control);
    k4 = nlf(0 + h, xk + h*k3, control);
    xk1 = xk + h/6*(k1 + 2*k2 + 2*k3 + k4);


    if dist
        xk1(1)=pi+deg2rad(5);
        xk(1) =pi+deg2rad(5);
    end


    % % Forward Euler
    % xk1 = xk + h*nlf(0, xk, control);
    % Take out states of interest
    y = [xk(1); xk(3)];
end

== matlab function reaction_pendulum_swingup/Pendulum nonlinear model2/Nonlinear dynamics ==
  data: H input; x0 input; control input; xp input; xk input size=[3,1]; xk1 output size=[3,1]; h parameter
function xk1   = nlrk4(H, x0, control, xp, xk, h)
    persistent initialized

    if isempty(initialized)
        xk1 = x0;
        theta_dd = 0;
        initialized = true;
        return;
    end

    function dx = nlf(t,x,u,xp,H)
        C = [1,0,0;0,0,1];

        % Define constants
        K1 = 10.6608;
        K2 = 0.0487;
        K3 = 0.1031;
        K4 = 404.3827;
        K5 = 0.9442;
        K6 = 1.7125;
        K_tau = 0.0107;
        
        % System equations
        theta = x(1);
        theta_dot = x(2);
        omega = x(3);
        theta_ddot = -K1*sin(theta)-K2*theta_dot-K3*sign(theta_dot)-K_tau*(K4*u-K5*omega-K6*sign(omega));
        omega_dot = K4*u-K5*omega-K6*sign(omega);
        delta = xp-C*x;
        Linear_term = H*(delta);
        NL_term = [theta_dot; theta_ddot; omega_dot] ;
        dx = NL_term + Linear_term;
    end

    function theta_ddot = theta_ddd(t,x,u,xp,H)
        C = [1,0,0;0,0,1];

        % Define constants
        K1 = 10.6608;
        K2 = 0.0487;
        K3 = 0.1031;
        K4 = 404.3827;
        K5 = 0.9442;
        K6 = 1.7125;
        K_tau = 0.0107;
        
        % System equations
        theta = x(1);
        theta_dot = x(2);
        omega = x(3);
        theta_ddot = -K1*sin(theta)-K2*theta_dot-K3*sign(theta_dot)-K_tau*(K4*u-K5*omega-K6*sign(omega));
    end

    theta_dd = theta_ddd(0, xk, control, xp, H);

    % Executes one timestep of the RK4 algorithm
    k1 = nlf(0, xk, control, xp, H);
    k2 = nlf(0 + h/2, xk + h/2*k1, control, xp + h/2*k1([1,3]), H);
    k3 = nlf(0 + h/2, xk + h/2*k2, control, xp + h/2*k2([1,3]), H);
    k4 = nlf(0 + h, xk + h*k3, control, xp + h*k3([1,3]), H);
    xk1 = xk + h/6*(k1 + 2*k2 + 2*k3 + k4);

    % % Forward Euler
    % xk1 = xk + h*nlf(0, xk, control);
    % Take out states of interest
    % y = [xk(1); xk(3)];
end

== matlab function reaction_pendulum_swingup/Pendulum nonlinear model1/Nonlinear dynamics ==
  data: x0 input; control input; xp input; H input; xk input size=[3,1]; xk1 output size=[3,1]; h parameter
function xk1   = nlrk4(x0, control, xp, H, xk, h)
    persistent initialized

    if isempty(initialized)
        xk1 = x0;
        theta_dd = 0;
        initialized = true;
        return;
    end

    function dx = nlf(t,x,u,xp,H)
        C = [1,0,0;0,0,1];

        % Define constants
        K1 = 10.6608;
        K2 = 0.0487;
        K3 = 0.1031;
        K4 = 404.3827;
        K5 = 0.9442;
        K6 = 1.7125;
        K_tau = 0.0107;
        
        % System equations
        theta = x(1);
        theta_dot = x(2);
        omega = x(3);
        theta_ddot = -K1*sin(theta)-K2*theta_dot-K3*sign(theta_dot)-K_tau*(K4*u-K5*omega-K6*sign(omega));
        omega_dot = K4*u-K5*omega-K6*sign(omega);
        delta = xp-C*x;
        Linear_term = H*(delta);
        NL_term = [theta_dot; theta_ddot; omega_dot] ;
        dx = NL_term + Linear_term;
    end

    function theta_ddot = theta_ddd(t,x,u,xp,H)
        C = [1,0,0;0,0,1];

        % Define constants
        K1 = 10.6608;
        K2 = 0.0487;
        K3 = 0.1031;
        K4 = 404.3827;
        K5 = 0.9442;
        K6 = 1.7125;
        K_tau = 0.0107;
        
        % System equations
        theta = x(1);
        theta_dot = x(2);
        omega = x(3);
        theta_ddot = -K1*sin(theta)-K2*theta_dot-K3*sign(theta_dot)-K_tau*(K4*u-K5*omega-K6*sign(omega));
    end

    theta_dd = theta_ddd(0, xk, control, xp, H);

    % Executes one timestep of the RK4 algorithm
    k1 = nlf(0, xk, control, xp, H);
    k2 = nlf(0 + h/2, xk + h/2*k1, control, xp + h/2*k1([1,3]), H);
    k3 = nlf(0 + h/2, xk + h/2*k2, control, xp + h/2*k2([1,3]), H);
    k4 = nlf(0 + h, xk + h*k3, control, xp + h*k3([1,3]), H);
    xk1 = xk + h/6*(k1 + 2*k2 + 2*k3 + k4);

    % % Forward Euler
    % xk1 = xk + h*nlf(0, xk, control);
    % Take out states of interest
    % y = [xk(1); xk(3)];
end
